simulink model "scope_test2"  (R2014a)
settings: Solver=ode45  StartTime=0.0  StopTime=2.0  FixedStep=0.5  RelTol=1e-3
settings Model: Creator=yangg  LastModifiedBy=yangg
settings DataIOCC: ExternalInput=[t', u']  SaveFormat=StructureWithTime  InspectSignalLogs=on  SaveTime=off
settings DebuggingCC: SolverPrmCheckMsg=none

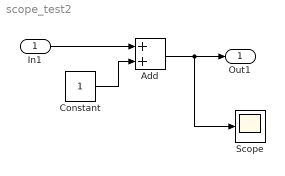
== system scope_test2 ==
  In1 : Inport
  Add : Sum
  Constant : Constant
  Scope : Scope
  Out1 : Outport
  wires:
  Add/1 -> Scope/1, Out1/1
  In1/1 -> Add/1
  Constant/1 -> Add/2
